simulink model "Planta_completa_controle_de_corrente"  (R2024a)
settings: Solver=FixedStepAuto  StartTime=0.0  StopTime=7  FixedStep=T  RelTol=1e-3
model workspace (MAT data in the model file):
  B = 0.0928996133407
  Cmn = 479.991198073
  I = 3000
  Ian = 260.13143483
  J = 0.56
  Kf = 1.91586963478
  La = 0.0014
  N = 3000
  Pele = 104052.573932
  Pmec = 95000
  Ra = 0.08
  T = 0.00175
  Te = 0.0175
  Tm = 6.02801217209
  Vn = 400
  Wn = 197.920296
libraries: simulink x3
settings Model: Creator=lpds  LastModifiedBy=lpds
settings RTWCC: GPUComputeCapability=3.5

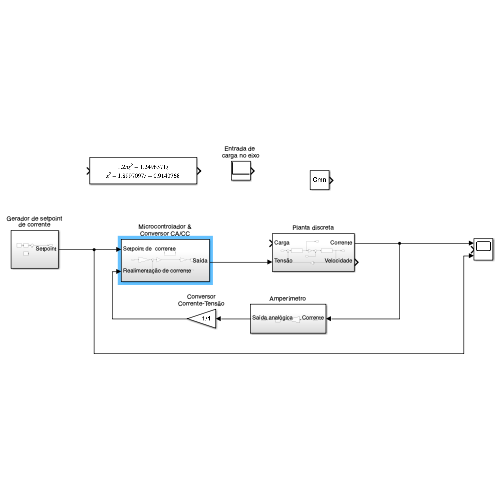
[thumbnail: Simulink's stored preview of the top-level diagram]
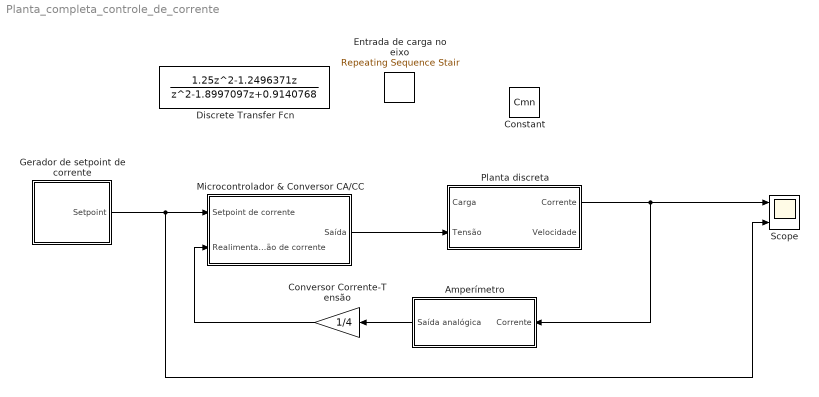
== system Planta_completa_controle_de_corrente ==
  Amperímetro : Subsystem
  Constant : Constant  Value=Cmn
  Conversor Corrente-Tensão : Gain  Gain=1/4
  Discrete Transfer Fcn : DiscreteTransferFcn  Numerator=[1.25, -1.2496371, 0]  Denominator=[1, -1.8997097, 0.9140768]
  Entrada de carga no eixo : simulink/Sources/Repeating Sequence Stair  OutValues=[Cmn]  tsamp=5000 * 0.00175  OutMin=[]  OutMax=[]  OutDataTypeStr=double  OutputDataTypeScalingMode=double  OutDataType=fixdt(0,8)  ConRadixGroup=Best Precision: Vector-wise  OutScaling=2^-12
  Gerador de setpoint de corrente : Subsystem
  Microcontrolador & Conversor CA/CC : Subsystem
  Planta discreta : Subsystem
  Scope : Scope  NumInputPorts=3
  wires:
  Conversor Corrente-Tensão/1 -> Microcontrolador & Conversor CA/CC/2(Realimentação de corrente)
  Amperímetro/1(Saída analógica) -> Conversor Corrente-Tensão/1
  Gerador de setpoint de corrente/1(Setpoint) -> Scope/3, Microcontrolador & Conversor CA/CC/1(Setpoint de corrente)
  Microcontrolador & Conversor CA/CC/1(Saída) -> Planta discreta/2(Tensão)
  Planta discreta/1(Corrente) -> Amperímetro/1(Corrente), Scope/1

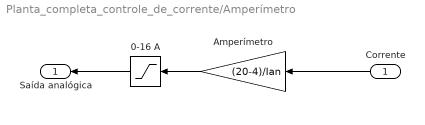
== system Planta_completa_controle_de_corrente/Amperímetro ==
  Corrente : Inport
  0-16 A : Saturate  UpperLimit=16  LowerLimit=0
  Amperímetro : Gain  Gain=(20-4)/Ian
  Saída analógica : Outport
  wires:
  Corrente/1 -> Amperímetro/1
  Amperímetro/1 -> 0-16 A/1
  0-16 A/1 -> Saída analógica/1

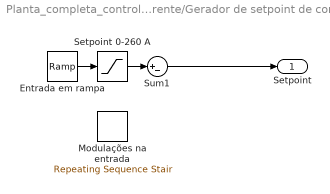
== system Planta_completa_controle_de_corrente/Gerador de setpoint de corrente ==
  Entrada em rampa : simulink/Sources/Ramp  slope=Ian*10  start=0  InitialOutput=0
  Modulações na entrada : simulink/Sources/Repeating Sequence Stair  OutValues=[0 50 -50].'  tsamp=1143 * 0.00175  OutMin=[]  OutMax=[]  OutDataTypeStr=double  OutputDataTypeScalingMode=double  OutDataType=fixdt(0,8)  ConRadixGroup=Best Precision: Vector-wise  OutScaling=2^-12
  Setpoint 0-260 A : Saturate  UpperLimit=10  LowerLimit=0
  Sum1 : Sum  Inputs=|+-
  Setpoint : Outport
  wires:
  Sum1/1 -> Setpoint/1
  Entrada em rampa/1 -> Setpoint 0-260 A/1
  Setpoint 0-260 A/1 -> Sum1/1

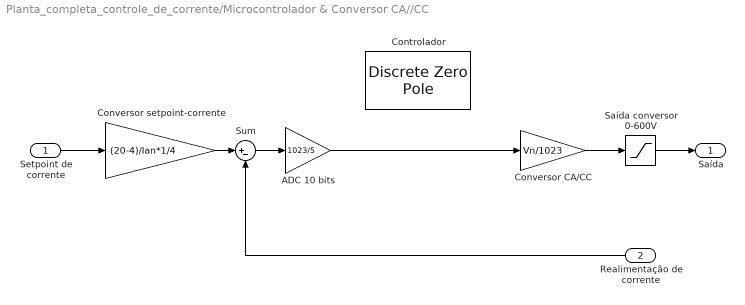
== system Planta_completa_controle_de_corrente/Microcontrolador & Conversor CA//CC ==
  Setpoint de corrente : Inport
  Realimentação de corrente : Inport  Port=2
  "ADC 10 bits " : Gain  Gain=1023/5
  Controlador : DiscreteZeroPole  Zeros=[0.9, 0.9]  Poles=[0, 1]  Gain=0.6  SampleTime=T
  Conversor setpoint-corrente : Gain  Gain=(20-4)/Ian*1/4
  Conversor CA/CC : Gain  Gain=Vn/1023
  Saída conversor 0-600V : Saturate  UpperLimit=600  LowerLimit=0
  Sum : Sum  Inputs=|+-
  Saída : Outport
  wires:
  Realimentação de corrente/1 -> Sum/2
  Sum/1 -> "ADC 10 bits "/1
  Conversor setpoint-corrente/1 -> Sum/1
  Saída conversor 0-600V/1 -> Saída/1
  Setpoint de corrente/1 -> Conversor setpoint-corrente/1
  Conversor CA/CC/1 -> Saída conversor 0-600V/1
  "ADC 10 bits "/1 -> Conversor CA/CC/1

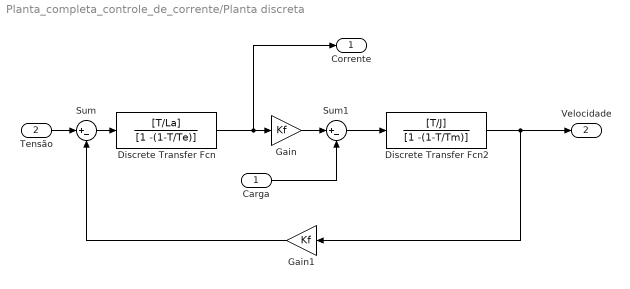
== system Planta_completa_controle_de_corrente/Planta discreta ==
  Carga : Inport
  Tensão : Inport  Port=2
  Discrete Transfer Fcn : DiscreteTransferFcn  Numerator=[T/La]  Denominator=[1 -(1-T/Te)]
  Discrete Transfer Fcn2 : DiscreteTransferFcn  Numerator=[T/J]  Denominator=[1 -(1-T/Tm)]
  Gain : Gain  Gain=Kf
  Gain1 : Gain  Gain=Kf
  Sum : Sum  Inputs=|+-
  Sum1 : Sum  Inputs=|+-
  Corrente : Outport
  Velocidade : Outport  Port=2
  wires:
  Gain/1 -> Sum1/1
  Gain1/1 -> Sum/2
  Sum/1 -> Discrete Transfer Fcn/1
  Carga/1 -> Sum1/2
  Discrete Transfer Fcn2/1 -> Velocidade/1, Gain1/1
  Sum1/1 -> Discrete Transfer Fcn2/1
  Tensão/1 -> Sum/1
  Discrete Transfer Fcn/1 -> Corrente/1, Gain/1
